simulink model "ACCMod002_dist"  (Simulink 8.3)
settings: Solver=ode45  StartTime=0.0  StopTime=10.0  RelTol=1e-3
model workspace (MAT data in the model file):
  pACC.Kp = 0.5
  pACC.minDist2Target = 50
  pACC.avgACCactiveTime = 20
  pACC.LearnGain = 0
  pACC.Ki = 1e-05
  pACC.KpDist = 1
  pACC.KiDist : numeric (value not decoded)
settings Model: Creator=swami  LastModifiedBy=swami
settings SolverCC: AutoInsertRateTranBlk=on
settings DataIOCC: SignalLoggingSaveFormat=Dataset
settings DebuggingCC: UnderspecifiedInitializationDetection=Simplified  StateNameClashWarn=none
settings GRTTargetCC: CombineOutputUpdateFcns=on  GRTInterface=off

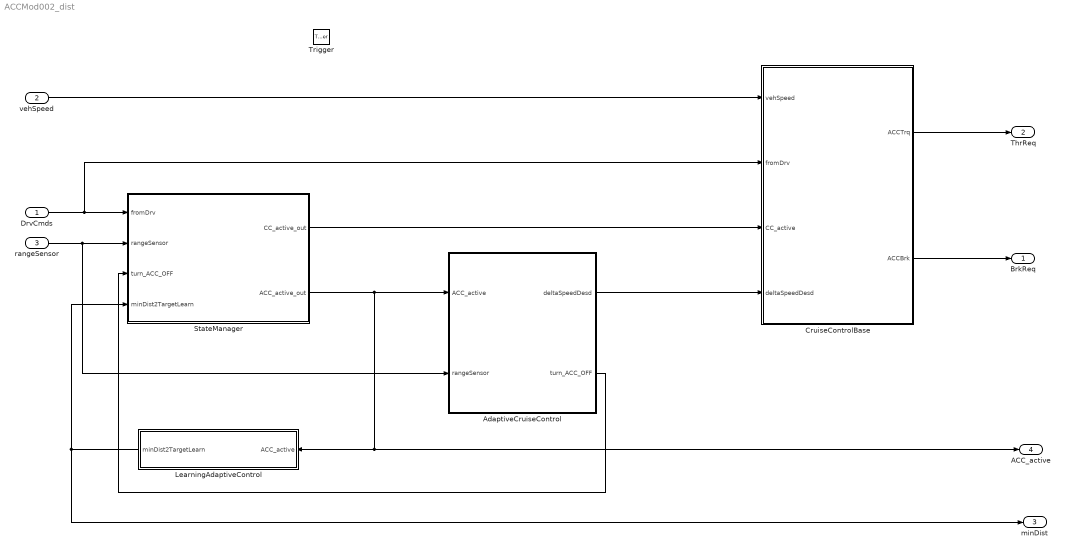
== system ACCMod002_dist ==
  DrvCmds : Inport  PortDimensions=4
  vehSpeed : Inport  Port=2
  rangeSensor : Inport  Port=3
  Trigger : TriggerPort  TriggerType=function-call  PortDimensions=1
  AdaptiveCruiseControl : MATLAB Function  TreatAsAtomicUnit=on
  CruiseControlBase : MATLAB Function  TreatAsAtomicUnit=on
  LearningAdaptiveControl : MATLAB Function  TreatAsAtomicUnit=on
  StateManager : MATLAB Function  TreatAsAtomicUnit=on
  BrkReq : Outport  PortDimensions=1  InitialOutput=0
  ThrReq : Outport  Port=2  PortDimensions=1  InitialOutput=0
  minDist : Outport  Port=3  PortDimensions=1  InitialOutput=50
  ACC_active : Outport  Port=4  PortDimensions=1  InitialOutput=0
  wires:
  StateManager/1(CC_active_out) -> CruiseControlBase/3(CC_active)
  AdaptiveCruiseControl/1(deltaSpeedDesd) -> CruiseControlBase/4(deltaSpeedDesd)
  StateManager/2(ACC_active_out) -> LearningAdaptiveControl/1(ACC_active), ACC_active/1, AdaptiveCruiseControl/1(ACC_active)
  DrvCmds/1 -> CruiseControlBase/2(fromDrv), StateManager/1(fromDrv)
  vehSpeed/1 -> CruiseControlBase/1(vehSpeed)
  rangeSensor/1 -> AdaptiveCruiseControl/2(rangeSensor), StateManager/2(rangeSensor)
  LearningAdaptiveControl/1(minDist2TargetLearn) -> minDist/1, StateManager/4(minDist2TargetLearn)
  AdaptiveCruiseControl/2(turn_ACC_OFF) -> StateManager/3(turn_ACC_OFF)
  CruiseControlBase/1(ACCTrq) -> ThrReq/1
  CruiseControlBase/2(ACCBrk) -> BrkReq/1

== matlab function StateManager ==
  data: CC_active_out output double; fromDrv input double; ACC_active_out output double; rangeSensor input double; turn_ACC_OFF input double; minDist2TargetLearn input double; pACC parameter double
function [CC_active_out,ACC_active_out] = fcn(fromDrv,rangeSensor,turn_ACC_OFF,minDist2TargetLearn, pACC)
%#codegen
persistent dbgcnt;
persistent CC_active;
persistent ACC_active;
if isempty(ACC_active)
    CC_active = 0;
    ACC_active = 0;
    dbgcnt = 0;
end
dbgcnt = dbgcnt + 1;

DrvCCSw = fromDrv(3);

dist2Target = rangeSensor(1);

minDist2Target = pACC.minDist2Target + minDist2TargetLearn;
ACCBuffer = minDist2Target * 0.9;
if DrvCCSw > 0.5
    if (CC_active == 0)
        CC_active = 1;
    end
    if (dist2Target < minDist2Target)
        % need to slow down
        ACC_active = 1;
    elseif (dist2Target > (minDist2Target + ACCBuffer))
        ACC_active = 0;
    end
    
    if (ACC_active == 1)            
        if turn_ACC_OFF > 0.5
            ACC_active = 0;
        end
    end
    
else
    CC_active = 0;
    ACC_active = 0;
end
ACC_active_out = ACC_active;
CC_active_out = CC_active;

== matlab function CruiseControlBase ==
  data: vehSpeed input double; fromDrv input double; CC_active input double; deltaSpeedDesd input double; ACCTrq output double; ACCBrk output double; pACC parameter double
function [ACCTrq,ACCBrk] = fcn(vehSpeed,fromDrv,CC_active,deltaSpeedDesd,pACC)
%#codegen
persistent torq_req_int;
persistent torq_req_old;
persistent CC_active_old;
if isempty(CC_active_old)    
    torq_req_int = 0;
    torq_req_old = 0;
end

DrvBrk = fromDrv(1);
DrvThr = fromDrv(2);
DrvCCSetPoint = fromDrv(4);

if CC_active > 0.5
        
   errorKp = (DrvCCSetPoint + deltaSpeedDesd - vehSpeed) * pACC.Kp;
   
   torq_req_int = torq_req_int + errorKp * pACC.Ki;    
   torq_req_prop = errorKp;   
   torq_req = torq_req_prop + torq_req_int;
   
   if (torq_req > 1.0)
       torq_req = 1.0;
   elseif (torq_req < -1.0)
       torq_req = -1.0;
   end    
   if torq_req < 0.0
       ACCBrk = 0.0 - torq_req;
       ACCTrq = 0.0;
   else
       ACCBrk = 0.0;
       ACCTrq = torq_req;
   end
else
    CC_active = 0;
    ACCTrq = DrvThr;
    ACCBrk = DrvBrk;
    torq_req = ACCTrq;
end
if ((CC_active_old ==0) && (CC_active == 1))
    torq_req_int = torq_req_old;
end

torq_req_old = torq_req;
CC_active_old = CC_active;

== matlab function AdaptiveCruiseControl ==
  data: ACC_active input double; rangeSensor input double; pACC parameter double; deltaSpeedDesd output double; turn_ACC_OFF output double
function [deltaSpeedDesd, turn_ACC_OFF]  = fcn(ACC_active,rangeSensor, pACC)
%#codegen
persistent ACC_active_old;
persistent errorKiDist;
if isempty(ACC_active_old)
    errorKiDist = 0;
end

dist2Target = rangeSensor(1);
minDist2Target = pACC.minDist2Target;
turn_ACC_OFF = 0;

if (ACC_active == 1)
    errorKpDist = (dist2Target - minDist2Target) * pACC.KpDist;
    errorKiDist = errorKiDist + errorKpDist * pACC.KiDist;
    deltaSpeedDesd = errorKpDist + errorKiDist;
    
    if deltaSpeedDesd > 0.0
        deltaSpeedDesd = 0;
        turn_ACC_OFF = 1;
    end

else
    deltaSpeedDesd = 0;
end
    
if ((ACC_active_old ==0) && (ACC_active == 1))
    errorKiDist = 0;
end
ACC_active_old = ACC_active;

== matlab function LearningAdaptiveControl ==
  settings: sampleTime=0.1
  data: ACC_active input double; minDist2TargetLearn output double; pACC parameter double
function minDist2TargetLearn  = fcn(ACC_active,pACC)
%#codegen
persistent ACC_active_old;
persistent ACC_starttime;
persistent intClk;
if isempty(ACC_active_old)
    ACC_active_old = ACC_active;
    minDist2TargetLearn = 0;
    ACC_starttime = 0; % would like to avaoid this
    intClk = 0;
end

SampleTime = 0.1;
intClk = intClk + SampleTime;
clktime = intClk;

if ((ACC_active_old == 0) && (ACC_active == 1))
    ACC_starttime = clktime;
end

%check if this is start of ACC turn off
if ((ACC_active_old == 1) && (ACC_active == 0))
    if (clktime - ACC_starttime) < pACC.avgACCactiveTime
        minDist2TargetLearn = minDist2TargetLearn + pACC.LearnGain;
    end
end

ACC_active_old = ACC_active;
